simulink model "PID_Continuous"  (R2018a)
settings: Solver=ode4  StartTime=0.0  StopTime=20  FixedStep=0.005  RelTol=1e-3
libraries: fuzblock x1
settings Model: SimulationMode=accelerator  Creator=dell  LastModifiedBy=dell

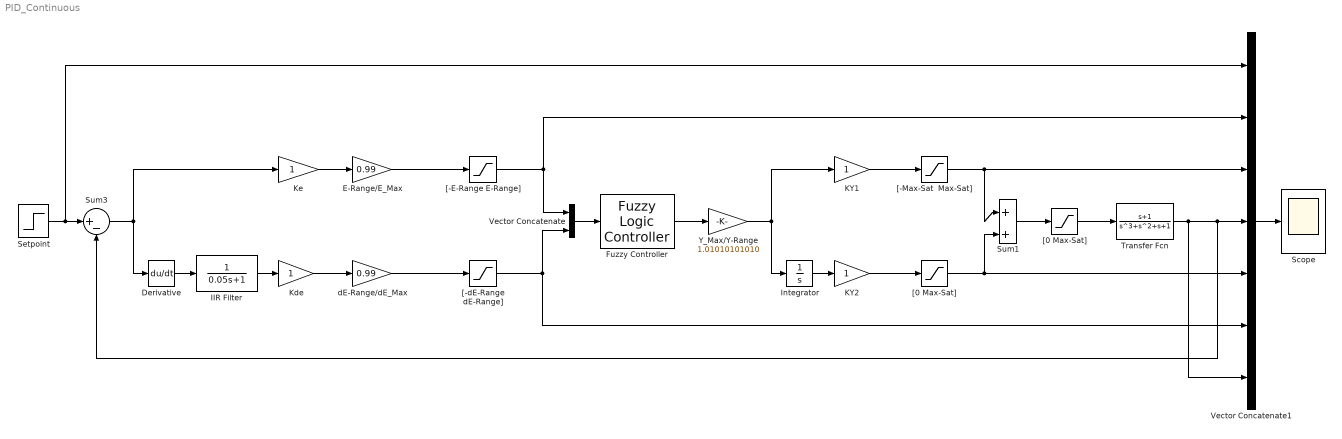
== system PID_Continuous ==
  "    Transfer Fcn   " : TransferFcn  Numerator=[1 1]  Denominator=[1 1 1 1]
  Derivative : Derivative
  E-Range/E_Max : Gain  Gain=0.99
  Fuzzy Controller : fuzblock/Fuzzy Logic  Controller  FIS='4.fis'  OutputSampleNumber=10  DataType=double  FuzzifiedInputs=off  RuleFiringStrengths=off  RuleOutputs=off  AggregatedOutputs=off  SimulateUsing=Interpreted execution  OutOfRangeInputValueMessage=none  NoRuleFiredMessage=none  EmptyOutputFuzzySetMessage=none
  IIR Filter : TransferFcn  Denominator=[0.05 1]
  Integrator : Integrator
  "KY1 " : Gain
  "KY2 " : Gain
  "Kde " : Gain
  "Ke " : Gain
  "Scope " : Scope
  "Setpoint " : Step  Time=0  After=50  SampleTime=0  VectorParams1D=off
  Sum1 : Sum  Inputs=|++
  Sum3 : Sum  Inputs=|+-
  Vector Concatenate : Concatenate
  Vector Concatenate1 : Concatenate  NumInputs=7
  "Y_Max/Y-Range " : Gain  Gain=1.01010101010
  "[-E-Range E-Range] " : Saturate  UpperLimit=99  LowerLimit=-99  LinearizeAsGain=off  OutMin=[-100]  OutMax=[100]
  "[-Max-Sat  Max-Sat] " : Saturate  UpperLimit=100  LowerLimit=-100  LinearizeAsGain=off
  "[-dE-Range dE-Range] " : Saturate  UpperLimit=99  LowerLimit=-99  LinearizeAsGain=off
  "[0 Max-Sat] " : Saturate  UpperLimit=100  LowerLimit=0  LinearizeAsGain=off
  "[0 Max-Sat] " : Saturate  UpperLimit=100  LowerLimit=0  LinearizeAsGain=off
  "dE-Range/dE_Max " : Gain  Gain=0.99
  wires:
  "[-dE-Range dE-Range] "/1 -> Vector Concatenate1/6, Vector Concatenate/2
  Vector Concatenate1/1 -> "Scope "/1
  E-Range/E_Max/1 -> "[-E-Range E-Range] "/1
  "Ke "/1 -> E-Range/E_Max/1
  "    Transfer Fcn   "/1 -> Vector Concatenate1/7, Vector Concatenate1/4, Sum3/2
  "dE-Range/dE_Max "/1 -> "[-dE-Range dE-Range] "/1
  "Y_Max/Y-Range "/1 -> "KY1 "/1, Integrator/1
  Sum3/1 -> Derivative/1, "Ke "/1
  "Kde "/1 -> "dE-Range/dE_Max "/1
  "[0 Max-Sat] "/1 -> "    Transfer Fcn   "/1
  Fuzzy Controller/1 -> "Y_Max/Y-Range "/1
  "[-E-Range E-Range] "/1 -> Vector Concatenate1/2, Vector Concatenate/1
  Sum1/1 -> "[0 Max-Sat] "/1
  "KY1 "/1 -> "[-Max-Sat  Max-Sat] "/1
  "KY2 "/1 -> "[0 Max-Sat] "/1
  Integrator/1 -> "KY2 "/1
  "[0 Max-Sat] "/1 -> Vector Concatenate1/5, Sum1/2
  Derivative/1 -> IIR Filter/1
  "[-Max-Sat  Max-Sat] "/1 -> Vector Concatenate1/3, Sum1/1
  IIR Filter/1 -> "Kde "/1
  Vector Concatenate/1 -> Fuzzy Controller/1
  "Setpoint "/1 -> Vector Concatenate1/1, Sum3/1
